simulink model "Simulation1"  (R2024b)
settings: Solver=VariableStepAuto  StartTime=0.0  StopTime=30  RelTol=1e-3
values from neighbouring files (symbols this model uses):
  R = [cos(theta) -sin(theta) 0 ... (first row only)    [EMG_Signals.m]
libraries: vrlib x1
settings Model: PacingRate=2  Creator=alvinisac  LastModifiedBy=alvinisac

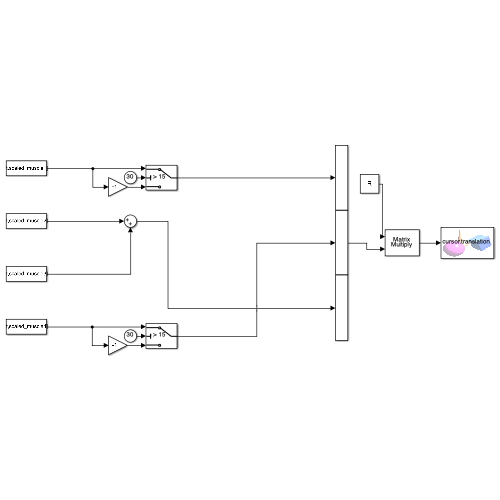
[thumbnail: Simulink's stored preview of the top-level diagram]
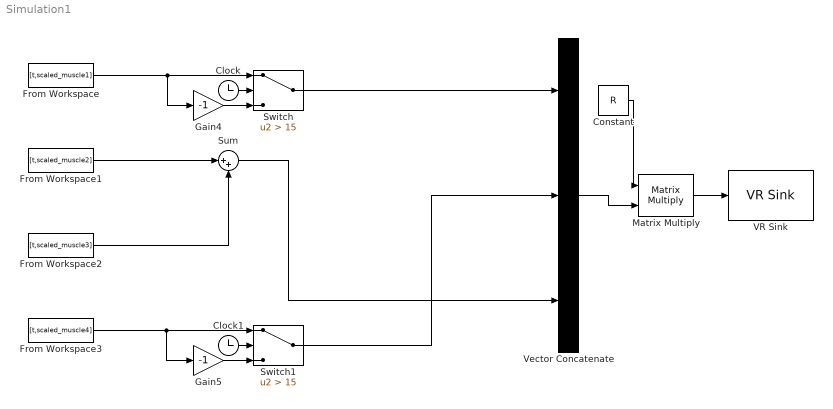
== system Simulation1 ==
  Clock : Clock
  Clock1 : Clock
  Constant : Constant  Value=R
  From Workspace : FromWorkspace  VariableName=[t,scaled_muscle1]
  From Workspace1 : FromWorkspace  VariableName=[t,scaled_muscle2]
  From Workspace2 : FromWorkspace  VariableName=[t,scaled_muscle3]
  From Workspace3 : FromWorkspace  VariableName=[t,scaled_muscle4]
  Gain4 : Gain  Gain=-1
  Gain5 : Gain  Gain=-1
  Matrix Multiply : Product  Multiplication=Matrix(*)
  Sum : Sum  Inputs=|++
  Switch : Switch  Criteria=u2 > Threshold  Threshold=15  SaturateOnIntegerOverflow=off  InputSameDT=off
  Switch1 : Switch  Criteria=u2 > Threshold  Threshold=15  SaturateOnIntegerOverflow=off  InputSameDT=off
  VR Sink : vrlib/VR Sink  InstantiateOnLoad=on  SampleTime=0.1  ViewEnable=on  RemoteChange=off  RemoteView=off  FieldsWritten=cursor.translation.3.1.1.double  WorldFileName=8_palline_color.wrl  AutoView=off  VideoDimensions=[]  AllowVariableSize=off  FigureProperties="{'Position', 'Name', 'Viewpoint', 'CameraBound', 'CameraDirection', 'CameraPosition', 'CameraUpVector', 'ZoomFactor', 'Antialiasing', 'Headlight', 'Lighting', 'Sound', 'StatusBar', 'Stereo3D', 'Stereo3DCameraOffset', 'Stereo3DHIT', 'ToolBar', 'Textures', 'Transparency', 'Triad', 'Wireframe', 'NavZones', 'NavMode', 'NavSpeed', 'CaptureFileFormat', 'CaptureFileName', 'Record2DCompressMethod', 'Record2DCompressQuality', 'Record2D', 'Record2DFileName', 'Record2DFPS', 'NavPanel'; [1.0000000000000000e+00   1.0300000000000000e+02   1.4400000000000000e+03   7.4600000000000000e+02], '', '_untitled_1', 'on', [0.0000000000000000e+00   0.0000000000000000e+00  -1.0000000000000000e+00], [0.0000000000000000e+00   0.0000000000000000e+00   0.0000000000000000e+00], [0.0000000000000000e+00   1.0000000000000000e+00   0.0000000000000000e+00], [1.0000000000000000e+00], 'on', 'on', 'on', 'on', 'on', 'off', [1.0000000149011612e-01], [0.0000000000000000e+00], 'on', 'on', 'on', 'none', 'off', 'off', 'fly', 'normal', 'tif', '%f_anim_%n.tif', 'auto', [7.5000000000000000e+01], 'off', '%f_anim_%n.avi', 'auto', 'halfbar'}"
  Vector Concatenate : Concatenate  NumInputs=3
  wires:
  From Workspace/1 -> Gain4/1, Switch/1
  From Workspace2/1 -> Sum/2
  From Workspace1/1 -> Sum/1
  Clock/1 -> Switch/2
  Gain4/1 -> Switch/3
  Switch/1 -> Vector Concatenate/1
  Switch1/1 -> Vector Concatenate/2
  Gain5/1 -> Switch1/3
  Clock1/1 -> Switch1/2
  From Workspace3/1 -> Gain5/1, Switch1/1
  Sum/1 -> Vector Concatenate/3
  Vector Concatenate/1 -> Matrix Multiply/2
  Constant/1 -> Matrix Multiply/1
  Matrix Multiply/1 -> VR Sink/1
